simulink model "Control_system_SS"  (R2019a)
settings: Solver=FixedStepAuto  StartTime=0.0  StopTime=20  FixedStep=0.01  RelTol=1e-3
values from neighbouring files (symbols this model uses):
  K1 = acker(A1,B1,P1)    [Controller_system_SS.m]    (also in SS_controller_design.m)
  L1 = place(A1',C1',OP1)'    [Controller_system_SS.m]    (also in SS_controller_design.m)
undefined symbols (not defined in the file or in its folder): A1, B1, C1
settings Model: Creator=Tyson  LastModifiedBy=Tyson

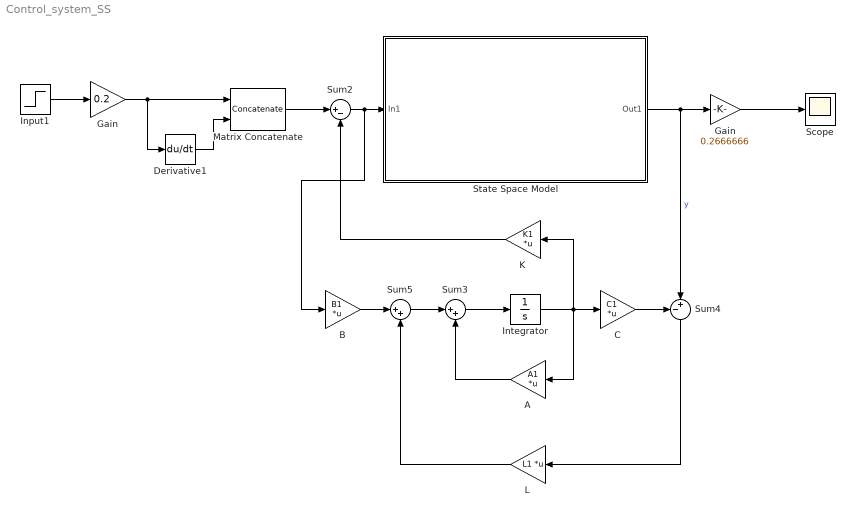
== system Control_system_SS ==
  "  A" : Gain  Gain=A1  Multiplication=Matrix(K*u)
  B : Gain  Gain=B1  Multiplication=Matrix(K*u)
  C : Gain  Gain=C1  Multiplication=Matrix(K*u)
  Derivative1 : Derivative
  Gain : Gain  Gain=0.2666666
  "Gain " : Gain  Gain=0.2
  Input1 : Step  After=5  SampleTime=0
  Integrator : Integrator
  K : Gain  Gain=K1  Multiplication=Matrix(K*u)
  L : Gain  Gain=L1  Multiplication=Matrix(K*u)
  Matrix Concatenate : Concatenate  Mode=Multidimensional array  ConcatenateDimension=2
  Scope : Scope
  State Space Model : Subsystem
  Sum2 : Sum  Inputs=|+-
  Sum3 : Sum  Inputs=|++
  Sum4 : Sum  Inputs=-+|
  Sum5 : Sum  Inputs=|++
  wires:
  Input1/1 -> "Gain "/1
  Derivative1/1 -> Matrix Concatenate/2
  State Space Model/1(Out1) -> Gain/1, Sum4/2  "y"
  Matrix Concatenate/1 -> Sum2/1
  Sum3/1 -> Integrator/1
  Integrator/1 -> C/1, "  A"/1, K/1
  K/1 -> Sum2/2
  Sum4/1 -> L/1
  "  A"/1 -> Sum3/2
  Sum5/1 -> Sum3/1
  L/1 -> Sum5/2
  C/1 -> Sum4/1
  B/1 -> Sum5/1
  "Gain "/1 -> Matrix Concatenate/1, Derivative1/1
  Sum2/1 -> B/1, State Space Model/1(In1)
  Gain/1 -> Scope/1

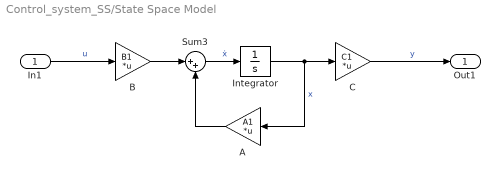
== system Control_system_SS/State Space Model ==
  In1 : Inport
  A : Gain  Gain=A1  Multiplication=Matrix(K*u)
  B : Gain  Gain=B1  Multiplication=Matrix(K*u)
  C : Gain  Gain=C1  Multiplication=Matrix(K*u)
  Integrator : Integrator
  Sum3 : Sum  Inputs=|++
  Out1 : Outport
  wires:
  In1/1 -> B/1  "u"
  B/1 -> Sum3/1
  A/1 -> Sum3/2
  Sum3/1 -> Integrator/1  "ẋ"
  C/1 -> Out1/1  "y"
  Integrator/1 -> C/1, A/1  "x"
